simulink model "BergmanModel_VaryingPulseLength"  (R2018b)
settings: Solver=VariableStepAuto  StartTime=0.0  StopTime=500  RelTol=1e-3
model workspace (MAT data in the model file):
  U1 = 100
  u2 = 0
settings Model: Creator=marti  LastModifiedBy=marti

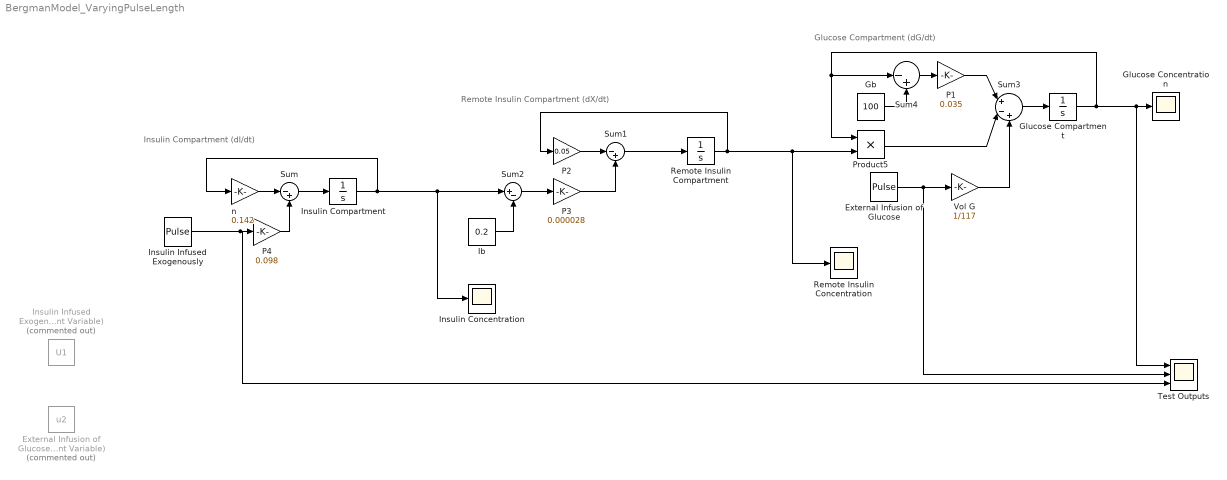
== system BergmanModel_VaryingPulseLength ==
  note: Insulin Compartment (dI/dt)
  note: Glucose Compartment (dG/dt)
  note: Remote Insulin Compartment (dX/dt)
  External Infusion of Glucose : DiscretePulseGenerator  PulseType=Time based  Amplitude=2  Period=195  PulseWidth=15  PhaseDelay=15
  External Infusion of Glucose (Constant Variable) : Constant  Commented=on  Value=u2
  Gb : Constant  Value=100
  Glucose Compartment : Integrator  InitialCondition=100
  Glucose Concentration : Scope
  Ib : Constant  Value=0.2
  Insulin Compartment : Integrator
  Insulin Concentration : Scope
  Insulin Infused Exogenously : DiscretePulseGenerator  PulseType=Time based  Amplitude=10  Period=195  PulseWidth=15
  Insulin Infused Exogenously (Constant Variable) : Constant  Commented=on  Value=U1  OutMin=0  OutMax=1000
  P1 : Gain  Gain=0.035
  P2 : Gain  Gain=0.05
  P3 : Gain  Gain=0.000028
  P4 : Gain  Gain=0.098
  Product5 : Product
  Remote Insulin Compartment : Integrator
  Remote Insulin Concentration : Scope
  Sum : Sum  Inputs=|-+
  Sum1 : Sum  Inputs=|-+
  Sum2 : Sum  Inputs=|+-
  Sum3 : Sum  Inputs=|+-+
  Sum4 : Sum  Inputs=|-+
  "Test Outputs " : Scope  NumInputPorts=3
  Vol G : Gain  Gain=1/117
  n : Gain  Gain=0.142
  wires:
  Remote Insulin Compartment/1 -> P2/1, Remote Insulin Concentration/1, Product5/2
  Insulin Compartment/1 -> n/1, Insulin Concentration/1, Sum2/1
  Product5/1 -> Sum3/2
  n/1 -> Sum/1
  P3/1 -> Sum1/2
  Sum1/1 -> Remote Insulin Compartment/1
  Gb/1 -> Sum4/2
  Sum/1 -> Insulin Compartment/1
  P2/1 -> Sum1/1
  Sum3/1 -> Glucose Compartment/1
  P1/1 -> Sum3/1
  Sum4/1 -> P1/1
  P4/1 -> Sum/2
  Glucose Compartment/1 -> Product5/1, Sum4/1, Glucose Concentration/1, "Test Outputs "/1
  Ib/1 -> Sum2/2
  Sum2/1 -> P3/1
  Vol G/1 -> Sum3/3
  Insulin Infused Exogenously/1 -> "Test Outputs "/3, P4/1
  External Infusion of Glucose/1 -> Vol G/1, "Test Outputs "/2
